simulink model "gm_parallel_min_cost_function_vopt_6phase"  (R2022a)
settings: Solver=FixedStepDiscrete  StartTime=0.0  StopTime=10.0  RelTol=1e-3
undefined symbols (not defined in the file or in its folder): f_c
libraries: hdlmdlgenlib x80
(part 2 of 3)

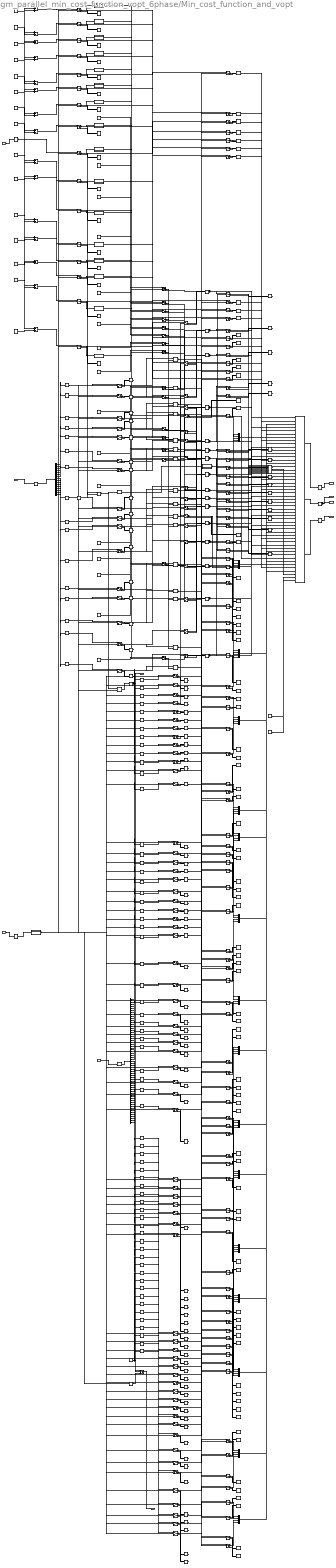
== system gm_parallel_min_cost_function_vopt_6phase/Min_cost_function_and_vopt ==
  Index_in : Inport  OutDataTypeStr=int32  PortDimensions=1  SampleTime=1e-08
  valid_in : Inport  Port=2  OutDataTypeStr=boolean  PortDimensions=1  SampleTime=1e-08
  J_in : Inport  Port=3  OutDataTypeStr=fixdt(1, 20, 11)  PortDimensions=[16]  SampleTime=1e-08
  phase_voltages_per_switching_state_in : Inport  Port=4  OutDataTypeStr=fixdt(1, 24, 11)  PortDimensions=[64]  SampleTime=1e-08
  Add{,1..14} (15 alike) : Sum  AccumDataTypeStr=fixdt(1, 33, 0)  OutDataTypeStr=fixdt(1, 33, 0)  SampleTime=1e-08
  Compare To Constant : Subsystem  mask(Compare To Constant){relop=<=, const=double(1), OutDataTypeStr=boolean, ZeroCross=on}
      mask prompts: relop "Simulink:masks:Operator_MP"; const "Simulink:masks:ConstantValue_MP"; OutDataTypeStr "Simulink:masks:OutputDataType_MP"; ZeroCross "Simulink:masks:EnableZerocrossingDetection_MP"
      mask help: Simulink:masks:CompareToConstant_MD
      mask init:
      | OutDataTypeStr = 'boolean';
      | ZeroCross = 'on';
      | blkName = 'parallel_min_cost_function_vopt_6phase/Min_cost_function_and_vopt/Compare\nTo Constant';
      | const = double(1);
      | const_str = '1';
      | const_val = double(1);
      | relop = '<=';
      | setValue = 'boolean';
      | str = '<= 1';
      mask TypeOptions relop: == | ~= | < | <= | >= | >
      mask TypeOptions OutDataTypeStr: Simulink:masks:uint8 | Simulink:masks:boolean
      mask Callback ZeroCross: sl('zeroCrossEnable', gcbh);
      mask Display: disp(str)
  Compare To Constant1 : Subsystem  mask(Compare To Constant){relop=<=, const=double(5), OutDataTypeStr=boolean, ZeroCross=on}
      mask prompts: relop "Simulink:masks:Operator_MP"; const "Simulink:masks:ConstantValue_MP"; OutDataTypeStr "Simulink:masks:OutputDataType_MP"; ZeroCross "Simulink:masks:EnableZerocrossingDetection_MP"
      mask help: Simulink:masks:CompareToConstant_MD
      mask init:
      | OutDataTypeStr = 'boolean';
      | ZeroCross = 'on';
      | blkName = 'parallel_min_cost_function_vopt_6phase/Min_cost_function_and_vopt/Compare\nTo Constant1';
      | const = double(5);
      | const_str = '5';
      | const_val = double(5);
      | relop = '<=';
      | setValue = 'boolean';
      | str = '<= 5';
      mask TypeOptions relop: == | ~= | < | <= | >= | >
      mask TypeOptions OutDataTypeStr: Simulink:masks:uint8 | Simulink:masks:boolean
      mask Callback ZeroCross: sl('zeroCrossEnable', gcbh);
      mask Display: disp(str)
  Compare To Constant10 : Subsystem  mask(Compare To Constant){relop=<=, const=double(41), OutDataTypeStr=boolean, ZeroCross=on}
      mask prompts: relop "Simulink:masks:Operator_MP"; const "Simulink:masks:ConstantValue_MP"; OutDataTypeStr "Simulink:masks:OutputDataType_MP"; ZeroCross "Simulink:masks:EnableZerocrossingDetection_MP"
      mask help: Simulink:masks:CompareToConstant_MD
      mask init:
      | OutDataTypeStr = 'boolean';
      | ZeroCross = 'on';
      | blkName = 'parallel_min_cost_function_vopt_6phase/Min_cost_function_and_vopt/Compare\nTo Constant10';
      | const = double(41);
      | const_str = '41';
      | const_val = double(41);
      | relop = '<=';
      | setValue = 'boolean';
      | str = '<= 41';
      mask TypeOptions relop: == | ~= | < | <= | >= | >
      mask TypeOptions OutDataTypeStr: Simulink:masks:uint8 | Simulink:masks:boolean
      mask Callback ZeroCross: sl('zeroCrossEnable', gcbh);
      mask Display: disp(str)
  Compare To Constant11 : Subsystem  mask(Compare To Constant){relop=<=, const=double(45), OutDataTypeStr=boolean, ZeroCross=on}
      mask prompts: relop "Simulink:masks:Operator_MP"; const "Simulink:masks:ConstantValue_MP"; OutDataTypeStr "Simulink:masks:OutputDataType_MP"; ZeroCross "Simulink:masks:EnableZerocrossingDetection_MP"
      mask help: Simulink:masks:CompareToConstant_MD
      mask init:
      | OutDataTypeStr = 'boolean';
      | ZeroCross = 'on';
      | blkName = 'parallel_min_cost_function_vopt_6phase/Min_cost_function_and_vopt/Compare\nTo Constant11';
      | const = double(45);
      | const_str = '45';
      | const_val = double(45);
      | relop = '<=';
      | setValue = 'boolean';
      | str = '<= 45';
      mask TypeOptions relop: == | ~= | < | <= | >= | >
      mask TypeOptions OutDataTypeStr: Simulink:masks:uint8 | Simulink:masks:boolean
      mask Callback ZeroCross: sl('zeroCrossEnable', gcbh);
      mask Display: disp(str)
  Compare To Constant12 : Subsystem  mask(Compare To Constant){relop=<=, const=double(49), OutDataTypeStr=boolean, ZeroCross=on}
      mask prompts: relop "Simulink:masks:Operator_MP"; const "Simulink:masks:ConstantValue_MP"; OutDataTypeStr "Simulink:masks:OutputDataType_MP"; ZeroCross "Simulink:masks:EnableZerocrossingDetection_MP"
      mask help: Simulink:masks:CompareToConstant_MD
      mask init:
      | OutDataTypeStr = 'boolean';
      | ZeroCross = 'on';
      | blkName = 'parallel_min_cost_function_vopt_6phase/Min_cost_function_and_vopt/Compare\nTo Constant12';
      | const = double(49);
      | const_str = '49';
      | const_val = double(49);
      | relop = '<=';
      | setValue = 'boolean';
      | str = '<= 49';
      mask TypeOptions relop: == | ~= | < | <= | >= | >
      mask TypeOptions OutDataTypeStr: Simulink:masks:uint8 | Simulink:masks:boolean
      mask Callback ZeroCross: sl('zeroCrossEnable', gcbh);
      mask Display: disp(str)
  Compare To Constant13 : Subsystem  mask(Compare To Constant){relop=<=, const=double(53), OutDataTypeStr=boolean, ZeroCross=on}
      mask prompts: relop "Simulink:masks:Operator_MP"; const "Simulink:masks:ConstantValue_MP"; OutDataTypeStr "Simulink:masks:OutputDataType_MP"; ZeroCross "Simulink:masks:EnableZerocrossingDetection_MP"
      mask help: Simulink:masks:CompareToConstant_MD
      mask init:
      | OutDataTypeStr = 'boolean';
      | ZeroCross = 'on';
      | blkName = 'parallel_min_cost_function_vopt_6phase/Min_cost_function_and_vopt/Compare\nTo Constant13';
      | const = double(53);
      | const_str = '53';
      | const_val = double(53);
      | relop = '<=';
      | setValue = 'boolean';
      | str = '<= 53';
      mask TypeOptions relop: == | ~= | < | <= | >= | >
      mask TypeOptions OutDataTypeStr: Simulink:masks:uint8 | Simulink:masks:boolean
      mask Callback ZeroCross: sl('zeroCrossEnable', gcbh);
      mask Display: disp(str)
  Compare To Constant14 : Subsystem  mask(Compare To Constant){relop=<=, const=double(57), OutDataTypeStr=boolean, ZeroCross=on}
      mask prompts: relop "Simulink:masks:Operator_MP"; const "Simulink:masks:ConstantValue_MP"; OutDataTypeStr "Simulink:masks:OutputDataType_MP"; ZeroCross "Simulink:masks:EnableZerocrossingDetection_MP"
      mask help: Simulink:masks:CompareToConstant_MD
      mask init:
      | OutDataTypeStr = 'boolean';
      | ZeroCross = 'on';
      | blkName = 'parallel_min_cost_function_vopt_6phase/Min_cost_function_and_vopt/Compare\nTo Constant14';
      | const = double(57);
      | const_str = '57';
      | const_val = double(57);
      | relop = '<=';
      | setValue = 'boolean';
      | str = '<= 57';
      mask TypeOptions relop: == | ~= | < | <= | >= | >
      mask TypeOptions OutDataTypeStr: Simulink:masks:uint8 | Simulink:masks:boolean
      mask Callback ZeroCross: sl('zeroCrossEnable', gcbh);
      mask Display: disp(str)
  Compare To Constant15 : Subsystem  mask(Compare To Constant){relop=<=, const=double(61), OutDataTypeStr=boolean, ZeroCross=on}
      mask prompts: relop "Simulink:masks:Operator_MP"; const "Simulink:masks:ConstantValue_MP"; OutDataTypeStr "Simulink:masks:OutputDataType_MP"; ZeroCross "Simulink:masks:EnableZerocrossingDetection_MP"
      mask help: Simulink:masks:CompareToConstant_MD
      mask init:
      | OutDataTypeStr = 'boolean';
      | ZeroCross = 'on';
      | blkName = 'parallel_min_cost_function_vopt_6phase/Min_cost_function_and_vopt/Compare\nTo Constant15';
      | const = double(61);
      | const_str = '61';
      | const_val = double(61);
      | relop = '<=';
      | setValue = 'boolean';
      | str = '<= 61';
      mask TypeOptions relop: == | ~= | < | <= | >= | >
      mask TypeOptions OutDataTypeStr: Simulink:masks:uint8 | Simulink:masks:boolean
      mask Callback ZeroCross: sl('zeroCrossEnable', gcbh);
      mask Display: disp(str)
  Compare To Constant2 : Subsystem  mask(Compare To Constant){relop=<=, const=double(9), OutDataTypeStr=boolean, ZeroCross=on}
      mask prompts: relop "Simulink:masks:Operator_MP"; const "Simulink:masks:ConstantValue_MP"; OutDataTypeStr "Simulink:masks:OutputDataType_MP"; ZeroCross "Simulink:masks:EnableZerocrossingDetection_MP"
      mask help: Simulink:masks:CompareToConstant_MD
      mask init:
      | OutDataTypeStr = 'boolean';
      | ZeroCross = 'on';
      | blkName = 'parallel_min_cost_function_vopt_6phase/Min_cost_function_and_vopt/Compare\nTo Constant2';
      | const = double(9);
      | const_str = '9';
      | const_val = double(9);
      | relop = '<=';
      | setValue = 'boolean';
      | str = '<= 9';
      mask TypeOptions relop: == | ~= | < | <= | >= | >
      mask TypeOptions OutDataTypeStr: Simulink:masks:uint8 | Simulink:masks:boolean
      mask Callback ZeroCross: sl('zeroCrossEnable', gcbh);
      mask Display: disp(str)
  Compare To Constant3 : Subsystem  mask(Compare To Constant){relop=<=, const=double(13), OutDataTypeStr=boolean, ZeroCross=on}
      mask prompts: relop "Simulink:masks:Operator_MP"; const "Simulink:masks:ConstantValue_MP"; OutDataTypeStr "Simulink:masks:OutputDataType_MP"; ZeroCross "Simulink:masks:EnableZerocrossingDetection_MP"
      mask help: Simulink:masks:CompareToConstant_MD
      mask init:
      | OutDataTypeStr = 'boolean';
      | ZeroCross = 'on';
      | blkName = 'parallel_min_cost_function_vopt_6phase/Min_cost_function_and_vopt/Compare\nTo Constant3';
      | const = double(13);
      | const_str = '13';
      | const_val = double(13);
      | relop = '<=';
      | setValue = 'boolean';
      | str = '<= 13';
      mask TypeOptions relop: == | ~= | < | <= | >= | >
      mask TypeOptions OutDataTypeStr: Simulink:masks:uint8 | Simulink:masks:boolean
      mask Callback ZeroCross: sl('zeroCrossEnable', gcbh);
      mask Display: disp(str)
  Compare To Constant4 : Subsystem  mask(Compare To Constant){relop=<=, const=double(17), OutDataTypeStr=boolean, ZeroCross=on}
      mask prompts: relop "Simulink:masks:Operator_MP"; const "Simulink:masks:ConstantValue_MP"; OutDataTypeStr "Simulink:masks:OutputDataType_MP"; ZeroCross "Simulink:masks:EnableZerocrossingDetection_MP"
      mask help: Simulink:masks:CompareToConstant_MD
      mask init:
      | OutDataTypeStr = 'boolean';
      | ZeroCross = 'on';
      | blkName = 'parallel_min_cost_function_vopt_6phase/Min_cost_function_and_vopt/Compare\nTo Constant4';
      | const = double(17);
      | const_str = '17';
      | const_val = double(17);
      | relop = '<=';
      | setValue = 'boolean';
      | str = '<= 17';
      mask TypeOptions relop: == | ~= | < | <= | >= | >
      mask TypeOptions OutDataTypeStr: Simulink:masks:uint8 | Simulink:masks:boolean
      mask Callback ZeroCross: sl('zeroCrossEnable', gcbh);
      mask Display: disp(str)
  Compare To Constant5 : Subsystem  mask(Compare To Constant){relop=<=, const=double(21), OutDataTypeStr=boolean, ZeroCross=on}
      mask prompts: relop "Simulink:masks:Operator_MP"; const "Simulink:masks:ConstantValue_MP"; OutDataTypeStr "Simulink:masks:OutputDataType_MP"; ZeroCross "Simulink:masks:EnableZerocrossingDetection_MP"
      mask help: Simulink:masks:CompareToConstant_MD
      mask init:
      | OutDataTypeStr = 'boolean';
      | ZeroCross = 'on';
      | blkName = 'parallel_min_cost_function_vopt_6phase/Min_cost_function_and_vopt/Compare\nTo Constant5';
      | const = double(21);
      | const_str = '21';
      | const_val = double(21);
      | relop = '<=';
      | setValue = 'boolean';
      | str = '<= 21';
      mask TypeOptions relop: == | ~= | < | <= | >= | >
      mask TypeOptions OutDataTypeStr: Simulink:masks:uint8 | Simulink:masks:boolean
      mask Callback ZeroCross: sl('zeroCrossEnable', gcbh);
      mask Display: disp(str)
  Compare To Constant6 : Subsystem  mask(Compare To Constant){relop=<=, const=double(25), OutDataTypeStr=boolean, ZeroCross=on}
      mask prompts: relop "Simulink:masks:Operator_MP"; const "Simulink:masks:ConstantValue_MP"; OutDataTypeStr "Simulink:masks:OutputDataType_MP"; ZeroCross "Simulink:masks:EnableZerocrossingDetection_MP"
      mask help: Simulink:masks:CompareToConstant_MD
      mask init:
      | OutDataTypeStr = 'boolean';
      | ZeroCross = 'on';
      | blkName = 'parallel_min_cost_function_vopt_6phase/Min_cost_function_and_vopt/Compare\nTo Constant6';
      | const = double(25);
      | const_str = '25';
      | const_val = double(25);
      | relop = '<=';
      | setValue = 'boolean';
      | str = '<= 25';
      mask TypeOptions relop: == | ~= | < | <= | >= | >
      mask TypeOptions OutDataTypeStr: Simulink:masks:uint8 | Simulink:masks:boolean
      mask Callback ZeroCross: sl('zeroCrossEnable', gcbh);
      mask Display: disp(str)
  Compare To Constant7 : Subsystem  mask(Compare To Constant){relop=<=, const=double(29), OutDataTypeStr=boolean, ZeroCross=on}
      mask prompts: relop "Simulink:masks:Operator_MP"; const "Simulink:masks:ConstantValue_MP"; OutDataTypeStr "Simulink:masks:OutputDataType_MP"; ZeroCross "Simulink:masks:EnableZerocrossingDetection_MP"
      mask help: Simulink:masks:CompareToConstant_MD
      mask init:
      | OutDataTypeStr = 'boolean';
      | ZeroCross = 'on';
      | blkName = 'parallel_min_cost_function_vopt_6phase/Min_cost_function_and_vopt/Compare\nTo Constant7';
      | const = double(29);
      | const_str = '29';
      | const_val = double(29);
      | relop = '<=';
      | setValue = 'boolean';
      | str = '<= 29';
      mask TypeOptions relop: == | ~= | < | <= | >= | >
      mask TypeOptions OutDataTypeStr: Simulink:masks:uint8 | Simulink:masks:boolean
      mask Callback ZeroCross: sl('zeroCrossEnable', gcbh);
      mask Display: disp(str)
  Compare To Constant8 : Subsystem  mask(Compare To Constant){relop=<=, const=double(33), OutDataTypeStr=boolean, ZeroCross=on}
      mask prompts: relop "Simulink:masks:Operator_MP"; const "Simulink:masks:ConstantValue_MP"; OutDataTypeStr "Simulink:masks:OutputDataType_MP"; ZeroCross "Simulink:masks:EnableZerocrossingDetection_MP"
      mask help: Simulink:masks:CompareToConstant_MD
      mask init:
      | OutDataTypeStr = 'boolean';
      | ZeroCross = 'on';
      | blkName = 'parallel_min_cost_function_vopt_6phase/Min_cost_function_and_vopt/Compare\nTo Constant8';
      | const = double(33);
      | const_str = '33';
      | const_val = double(33);
      | relop = '<=';
      | setValue = 'boolean';
      | str = '<= 33';
      mask TypeOptions relop: == | ~= | < | <= | >= | >
      mask TypeOptions OutDataTypeStr: Simulink:masks:uint8 | Simulink:masks:boolean
      mask Callback ZeroCross: sl('zeroCrossEnable', gcbh);
      mask Display: disp(str)
  Compare To Constant9 : Subsystem  mask(Compare To Constant){relop=<=, const=double(37), OutDataTypeStr=boolean, ZeroCross=on}
      mask prompts: relop "Simulink:masks:Operator_MP"; const "Simulink:masks:ConstantValue_MP"; OutDataTypeStr "Simulink:masks:OutputDataType_MP"; ZeroCross "Simulink:masks:EnableZerocrossingDetection_MP"
      mask help: Simulink:masks:CompareToConstant_MD
      mask init:
      | OutDataTypeStr = 'boolean';
      | ZeroCross = 'on';
      | blkName = 'parallel_min_cost_function_vopt_6phase/Min_cost_function_and_vopt/Compare\nTo Constant9';
      | const = double(37);
      | const_str = '37';
      | const_val = double(37);
      | relop = '<=';
      | setValue = 'boolean';
      | str = '<= 37';
      mask TypeOptions relop: == | ~= | < | <= | >= | >
      mask TypeOptions OutDataTypeStr: Simulink:masks:uint8 | Simulink:masks:boolean
      mask Callback ZeroCross: sl('zeroCrossEnable', gcbh);
      mask Display: disp(str)
  Constant{,3..17} (16 alike) : Constant  Value=250  OutDataTypeStr=fixdt(1, 20, 11)  SampleTime=1e-08
  Constant1 : Constant  Value=4  OutDataTypeStr=int32  SampleTime=1e-08
  Constant18 : Constant  Value=4  OutDataTypeStr=int32  SampleTime=1e-08
  Constant19 : Constant  Value=8  OutDataTypeStr=int32  SampleTime=1e-08
  Constant2 : Constant  Value=0  OutDataTypeStr=boolean  SampleTime=1e-08
  Constant20 : Constant  Value=12  OutDataTypeStr=int32  SampleTime=1e-08
  Constant21 : Constant  Value=16  OutDataTypeStr=int32  SampleTime=1e-08
  Constant22 : Constant  Value=20  OutDataTypeStr=int32  SampleTime=1e-08
  Constant23 : Constant  Value=24  OutDataTypeStr=int32  SampleTime=1e-08
  Constant24 : Constant  Value=28  OutDataTypeStr=int32  SampleTime=1e-08
  Constant25 : Constant  Value=32  OutDataTypeStr=int32  SampleTime=1e-08
  Constant26 : Constant  Value=36  OutDataTypeStr=int32  SampleTime=1e-08
  Constant27 : Constant  Value=40  OutDataTypeStr=int32  SampleTime=1e-08
  Constant28 : Constant  Value=44  OutDataTypeStr=int32  SampleTime=1e-08
  Constant29 : Constant  Value=48  OutDataTypeStr=int32  SampleTime=1e-08
  Constant30 : Constant  Value=52  OutDataTypeStr=int32  SampleTime=1e-08
  Constant31 : Constant  Value=56  OutDataTypeStr=int32  SampleTime=1e-08
  Constant32 : Constant  Value=60  OutDataTypeStr=int32  SampleTime=1e-08
  Constant33 : Constant  Value=0  OutDataTypeStr=fixdt(1, 20, 11)  SampleTime=1e-08
  Constant34 : Constant  Value="repmat(0,[4  1])"  OutDataTypeStr=fixdt(1, 24, 11)  SampleTime=1e-08
  Delay{,1..5,7..8,12..22,25..26,34..43,46,49..50,58..67,72..73,81..90,95..96,104..113,118..119,127..136,141..142,150..159,164..165,173..182,191..200,205..206,214..223,228..229,237..246,251..252,260..269,274..275,283..292,297..298,302..303,311..320,325..326,334..343,348..349,357..366,371..386} (216 alike) : Delay  DelayLength=double(1)  InitialCondition=0  SampleTime=1e-08
  Delay16_out1_0_wire : hdlmdlgenlib/Buffer
      settings: SourceProductBaseCode=SL
  Delay16_out1_10_wire : hdlmdlgenlib/Buffer
      settings: SourceProductBaseCode=SL
  Delay16_out1_11_wire : hdlmdlgenlib/Buffer
      settings: SourceProductBaseCode=SL
  Delay16_out1_12_wire : hdlmdlgenlib/Buffer
      settings: SourceProductBaseCode=SL
  Delay16_out1_13_wire : hdlmdlgenlib/Buffer
      settings: SourceProductBaseCode=SL
  Delay16_out1_14_wire : hdlmdlgenlib/Buffer
      settings: SourceProductBaseCode=SL
  Delay16_out1_15_wire : hdlmdlgenlib/Buffer
      settings: SourceProductBaseCode=SL
  Delay16_out1_16_wire : hdlmdlgenlib/Buffer
      settings: SourceProductBaseCode=SL
  Delay16_out1_17_wire : hdlmdlgenlib/Buffer
      settings: SourceProductBaseCode=SL
  Delay16_out1_18_wire : hdlmdlgenlib/Buffer
      settings: SourceProductBaseCode=SL
  Delay16_out1_19_wire : hdlmdlgenlib/Buffer
      settings: SourceProductBaseCode=SL
  Delay16_out1_1_wire : hdlmdlgenlib/Buffer
      settings: SourceProductBaseCode=SL
  Delay16_out1_20_wire : hdlmdlgenlib/Buffer
      settings: SourceProductBaseCode=SL
  Delay16_out1_21_wire : hdlmdlgenlib/Buffer
      settings: SourceProductBaseCode=SL
  Delay16_out1_22_wire : hdlmdlgenlib/Buffer
      settings: SourceProductBaseCode=SL
  Delay16_out1_23_wire : hdlmdlgenlib/Buffer
      settings: SourceProductBaseCode=SL
  Delay16_out1_24_wire : hdlmdlgenlib/Buffer
      settings: SourceProductBaseCode=SL
  Delay16_out1_25_wire : hdlmdlgenlib/Buffer
      settings: SourceProductBaseCode=SL
  Delay16_out1_26_wire : hdlmdlgenlib/Buffer
      settings: SourceProductBaseCode=SL
  Delay16_out1_27_wire : hdlmdlgenlib/Buffer
      settings: SourceProductBaseCode=SL
  Delay16_out1_28_wire : hdlmdlgenlib/Buffer
      settings: SourceProductBaseCode=SL
  Delay16_out1_29_wire : hdlmdlgenlib/Buffer
      settings: SourceProductBaseCode=SL
  Delay16_out1_2_wire : hdlmdlgenlib/Buffer
      settings: SourceProductBaseCode=SL
  Delay16_out1_30_wire : hdlmdlgenlib/Buffer
      settings: SourceProductBaseCode=SL
  Delay16_out1_31_wire : hdlmdlgenlib/Buffer
      settings: SourceProductBaseCode=SL
  Delay16_out1_32_wire : hdlmdlgenlib/Buffer
      settings: SourceProductBaseCode=SL
  Delay16_out1_33_wire : hdlmdlgenlib/Buffer
      settings: SourceProductBaseCode=SL
  Delay16_out1_34_wire : hdlmdlgenlib/Buffer
      settings: SourceProductBaseCode=SL
  Delay16_out1_35_wire : hdlmdlgenlib/Buffer
      settings: SourceProductBaseCode=SL
  Delay16_out1_36_wire : hdlmdlgenlib/Buffer
      settings: SourceProductBaseCode=SL
  Delay16_out1_37_wire : hdlmdlgenlib/Buffer
      settings: SourceProductBaseCode=SL
  Delay16_out1_38_wire : hdlmdlgenlib/Buffer
      settings: SourceProductBaseCode=SL
  Delay16_out1_39_wire : hdlmdlgenlib/Buffer
      settings: SourceProductBaseCode=SL
  Delay16_out1_3_wire : hdlmdlgenlib/Buffer
      settings: SourceProductBaseCode=SL
  Delay16_out1_40_wire : hdlmdlgenlib/Buffer
      settings: SourceProductBaseCode=SL
  Delay16_out1_41_wire : hdlmdlgenlib/Buffer
      settings: SourceProductBaseCode=SL
  Delay16_out1_42_wire : hdlmdlgenlib/Buffer
      settings: SourceProductBaseCode=SL
  Delay16_out1_43_wire : hdlmdlgenlib/Buffer
      settings: SourceProductBaseCode=SL
  Delay16_out1_44_wire : hdlmdlgenlib/Buffer
      settings: SourceProductBaseCode=SL
  Delay16_out1_45_wire : hdlmdlgenlib/Buffer
      settings: SourceProductBaseCode=SL
  Delay16_out1_46_wire : hdlmdlgenlib/Buffer
      settings: SourceProductBaseCode=SL
  Delay16_out1_47_wire : hdlmdlgenlib/Buffer
      settings: SourceProductBaseCode=SL
  Delay16_out1_48_wire : hdlmdlgenlib/Buffer
      settings: SourceProductBaseCode=SL
  Delay16_out1_49_wire : hdlmdlgenlib/Buffer
      settings: SourceProductBaseCode=SL
  Delay16_out1_4_wire : hdlmdlgenlib/Buffer
      settings: SourceProductBaseCode=SL
  Delay16_out1_50_wire : hdlmdlgenlib/Buffer
      settings: SourceProductBaseCode=SL
  Delay16_out1_51_wire : hdlmdlgenlib/Buffer
      settings: SourceProductBaseCode=SL
  Delay16_out1_52_wire : hdlmdlgenlib/Buffer
      settings: SourceProductBaseCode=SL
  Delay16_out1_53_wire : hdlmdlgenlib/Buffer
      settings: SourceProductBaseCode=SL
  Delay16_out1_54_wire : hdlmdlgenlib/Buffer
      settings: SourceProductBaseCode=SL
  Delay16_out1_55_wire : hdlmdlgenlib/Buffer
      settings: SourceProductBaseCode=SL
  Delay16_out1_56_wire : hdlmdlgenlib/Buffer
      settings: SourceProductBaseCode=SL
  Delay16_out1_57_wire : hdlmdlgenlib/Buffer
      settings: SourceProductBaseCode=SL
  Delay16_out1_58_wire : hdlmdlgenlib/Buffer
      settings: SourceProductBaseCode=SL
  Delay16_out1_59_wire : hdlmdlgenlib/Buffer
      settings: SourceProductBaseCode=SL
  Delay16_out1_5_wire : hdlmdlgenlib/Buffer
      settings: SourceProductBaseCode=SL
  Delay16_out1_60_wire : hdlmdlgenlib/Buffer
      settings: SourceProductBaseCode=SL
  Delay16_out1_61_wire : hdlmdlgenlib/Buffer
      settings: SourceProductBaseCode=SL
  Delay16_out1_62_wire : hdlmdlgenlib/Buffer
      settings: SourceProductBaseCode=SL
  Delay16_out1_63_wire : hdlmdlgenlib/Buffer
      settings: SourceProductBaseCode=SL
  Delay16_out1_6_wire : hdlmdlgenlib/Buffer
      settings: SourceProductBaseCode=SL
  Delay16_out1_7_wire : hdlmdlgenlib/Buffer
      settings: SourceProductBaseCode=SL
  Delay16_out1_8_wire : hdlmdlgenlib/Buffer
      settings: SourceProductBaseCode=SL
  Delay16_out1_9_wire : hdlmdlgenlib/Buffer
      settings: SourceProductBaseCode=SL
  Delay23 : Delay  DelayLength=double(3)  InitialCondition=0  SampleTime=1e-08
  Delay24 : Delay  DelayLength=double(3)  InitialCondition=0  SampleTime=1e-08
  Delay7_out1_0_wire : hdlmdlgenlib/Buffer
      settings: SourceProductBaseCode=SL
  Delay7_out1_10_wire : hdlmdlgenlib/Buffer
      settings: SourceProductBaseCode=SL
  Delay7_out1_11_wire : hdlmdlgenlib/Buffer
      settings: SourceProductBaseCode=SL
  Delay7_out1_12_wire : hdlmdlgenlib/Buffer
      settings: SourceProductBaseCode=SL
  Delay7_out1_13_wire : hdlmdlgenlib/Buffer
      settings: SourceProductBaseCode=SL
  Delay7_out1_14_wire : hdlmdlgenlib/Buffer
      settings: SourceProductBaseCode=SL
  Delay7_out1_15_wire : hdlmdlgenlib/Buffer
      settings: SourceProductBaseCode=SL
  Delay7_out1_1_wire : hdlmdlgenlib/Buffer
      settings: SourceProductBaseCode=SL
  Delay7_out1_2_wire : hdlmdlgenlib/Buffer
      settings: SourceProductBaseCode=SL
  Delay7_out1_3_wire : hdlmdlgenlib/Buffer
      settings: SourceProductBaseCode=SL
  Delay7_out1_4_wire : hdlmdlgenlib/Buffer
      settings: SourceProductBaseCode=SL
  Delay7_out1_5_wire : hdlmdlgenlib/Buffer
      settings: SourceProductBaseCode=SL
  Delay7_out1_6_wire : hdlmdlgenlib/Buffer
      settings: SourceProductBaseCode=SL
  Delay7_out1_7_wire : hdlmdlgenlib/Buffer
      settings: SourceProductBaseCode=SL
  Delay7_out1_8_wire : hdlmdlgenlib/Buffer
      settings: SourceProductBaseCode=SL
  Delay7_out1_9_wire : hdlmdlgenlib/Buffer
      settings: SourceProductBaseCode=SL
  Detect Rise Positive : Subsystem  mask(Detect Rise Positive){vinit=double(0), InputProcessing=Elements as channels (sample based), OutDataTypeStr=boolean}
      mask prompts: vinit "Simulink:masks:InitialCondition_MP"; InputProcessing "Simulink:masks:InputProcessing_MP"; OutDataTypeStr "Simulink:masks:OutputDataType_MP"
      mask help: Simulink:masks:DetectRisePositive_MD
      mask init:
      | InputProcessing = 'Elements as channels (sample based)';
      | OutDataTypeStr = 'boolean';
      | vinit = double(0);
      mask TypeOptions InputProcessing: Simulink:masks:ColumnsAsChannelsFrameBased | Simulink:masks:ElementsAsChannelsSampleBased
      mask TypeOptions OutDataTypeStr: Simulink:masks:uint8 | Simulink:masks:boolean
      mask Display: fprintf('U > 0\n&  NOT\nU/z > 0')
  Detect Rise Positive1 : Subsystem  mask(Detect Rise Positive){vinit=double(0), InputProcessing=Elements as channels (sample based), OutDataTypeStr=boolean}
      mask prompts: vinit "Simulink:masks:InitialCondition_MP"; InputProcessing "Simulink:masks:InputProcessing_MP"; OutDataTypeStr "Simulink:masks:OutputDataType_MP"
      mask help: Simulink:masks:DetectRisePositive_MD
      mask init:
      | InputProcessing = 'Elements as channels (sample based)';
      | OutDataTypeStr = 'boolean';
      | vinit = double(0);
      mask TypeOptions InputProcessing: Simulink:masks:ColumnsAsChannelsFrameBased | Simulink:masks:ElementsAsChannelsSampleBased
      mask TypeOptions OutDataTypeStr: Simulink:masks:uint8 | Simulink:masks:boolean
      mask Display: fprintf('U > 0\n&  NOT\nU/z > 0')
  Logical Operator : Logic  AllPortsSameDT=off  OutDataTypeStr=boolean  SampleTime=1e-08
  MATLAB Function : Subsystem
  MinMax : MinMax  Inputs=16
  Relational Operator{,2..16} (16 alike) : RelationalOperator  Operator=<=  OutDataTypeStr=boolean  SampleTime=1e-08  InputSameDT=off
  Relational Operator1 : RelationalOperator  Operator===  OutDataTypeStr=boolean  SampleTime=1e-08  InputSameDT=off
  Switch{,1,8..9,20..21,27..28,34..35,41..42,48..49,55..56,62..63,69..70,76..77,83..84,90..91,97..98,104..105,111..112} (32 alike) : Switch  Criteria=u2 > Threshold  Threshold=double(0)  OutDataTypeStr=fixdt(1, 20, 11)  SampleTime=1e-08  SaturateOnIntegerOverflow=off  InputSameDT=off
  Switch{2,10,15,22,29,36,43,50,57,64,71,78,85,92,99,106} (16 alike) : Switch  Criteria=u2 > Threshold  Threshold=double(0)  OutDataTypeStr=int32  SampleTime=1e-08  SaturateOnIntegerOverflow=off  InputSameDT=off
  Switch{3..6,11..14,16..19,23..26,30..33,37..40,44..47,51..54,58..61,65..68,72..75,79..82,86..89,93..96,100..103,107..110} (64 alike) : Switch  Criteria=u2 > Threshold  Threshold=double(0)  OutDataTypeStr=fixdt(1, 24, 11)  SampleTime=1e-08  SaturateOnIntegerOverflow=off  InputSameDT=off
  Switch7 : Switch  Criteria=u2 > Threshold  Threshold=double(0)  OutDataTypeStr=boolean  SampleTime=1e-08  SaturateOnIntegerOverflow=off  InputSameDT=off
  Switch_on1 : Switch  Threshold=double(1)  OutDataTypeStr=int32  RndMeth=Simplest  SampleTime=1e-08  SaturateOnIntegerOverflow=off  InputSameDT=off
  Switch_on{4,10,14,20,26,32,38,44,50,56,62,68,74,80,86,92,98..113} (32 alike) : Switch  Threshold=double(1)  OutDataTypeStr=fixdt(1, 20, 11)  RndMeth=Simplest  SampleTime=1e-08  SaturateOnIntegerOverflow=off  InputSameDT=off
  Switch_on{2..3,5..6,8..9,11..12,15..16,18..19,21..22,24..25,27..28,30..31,33..34,36..37,39..40,42..43,45..46,48..49,51..52,54..55,57..58,60..61,63..64,66..67,69..70,72..73,75..76,78..79,81..82,84..85,87..88,90..91,93..94,96..97} (64 alike) : Switch  Threshold=double(1)  OutDataTypeStr=fixdt(1, 24, 11)  RndMeth=Simplest  SampleTime=1e-08  SaturateOnIntegerOverflow=off  InputSameDT=off
  Switch_on{7,17,23,29,35,41,47,53,59,65,71,77,83,89,95} (15 alike) : Switch  Threshold=double(1)  OutDataTypeStr=fixdt(1, 33, 0)  RndMeth=Simplest  SampleTime=1e-08  SaturateOnIntegerOverflow=off  InputSameDT=off
  mux{,1..15} (16 alike) : Mux
  t : Demux  Outputs=16
  t1 : Demux  Outputs=64
  done : Outport  SampleTime=1e-08
  done_complete : Outport  Port=2  SampleTime=1e-08
  J_AXI : Outport  Port=3  SampleTime=1e-08
  Index : Outport  Port=4  SampleTime=1e-08
  voltages : Outport  Port=5  SampleTime=1e-08
  Index_AXI : Outport  Port=6  SampleTime=1e-08
  wires:
  Index_in/1 -> Delay8/1
  valid_in/1 -> Delay46/1
  J_in/1 -> Delay7/1
  phase_voltages_per_switching_state_in/1 -> Delay16/1
  Add/1 -> Switch_on7/1
  Add1/1 -> Switch_on17/1
  Add10/1 -> Switch_on71/1
  Add11/1 -> Switch_on77/1
  Add12/1 -> Switch_on83/1
  Add13/1 -> Switch_on89/1
  Add14/1 -> Switch_on95/1
  Add2/1 -> Switch_on23/1
  Add3/1 -> Switch_on29/1
  Add4/1 -> Switch_on35/1
  Add5/1 -> Switch_on41/1
  Add6/1 -> Switch_on47/1
  Add7/1 -> Switch_on53/1
  Add8/1 -> Switch_on59/1
  Add9/1 -> Switch_on65/1
  Compare To Constant/1(y) -> Switch/2
  Compare To Constant1/1(y) -> Switch8/2
  Compare To Constant10/1(y) -> Switch76/2
  Compare To Constant11/1(y) -> Switch83/2
  Compare To Constant12/1(y) -> Switch90/2
  Compare To Constant13/1(y) -> Switch97/2
  Compare To Constant14/1(y) -> Switch104/2
  Compare To Constant15/1(y) -> Switch111/2
  Compare To Constant2/1(y) -> Switch20/2
  Compare To Constant3/1(y) -> Switch27/2
  Compare To Constant4/1(y) -> Switch34/2
  Compare To Constant5/1(y) -> Switch41/2
  Compare To Constant6/1(y) -> Switch48/2
  Compare To Constant7/1(y) -> Switch55/2
  Compare To Constant8/1(y) -> Switch62/2
  Compare To Constant9/1(y) -> Switch69/2
  Constant/1 -> Switch/1
  Constant1/1 -> Relational Operator1/1
  Constant10/1 -> Switch62/1
  Constant11/1 -> Switch69/1
  Constant12/1 -> Switch76/1
  Constant13/1 -> Switch83/1
  Constant14/1 -> Switch90/1
  Constant15/1 -> Switch97/1
  Constant16/1 -> Switch104/1
  Constant17/1 -> Switch111/1
  Constant18/1 -> Add/2
  Constant19/1 -> Add1/2
  Constant2/1 -> Switch7/1
  Constant20/1 -> Add2/2
  Constant21/1 -> Add3/2
  Constant22/1 -> Add4/2
  Constant23/1 -> Add5/2
  Constant24/1 -> Add6/2
  Constant25/1 -> Add7/2
  Constant26/1 -> Add8/2
  Constant27/1 -> Add9/2
  Constant28/1 -> Add10/2
  Constant29/1 -> Add11/2
  Constant3/1 -> Switch8/1
  Constant30/1 -> Add12/2
  Constant31/1 -> Add13/2
  Constant32/1 -> Add14/2
  Constant33/1 -> MATLAB Function/50(J_default)
  Constant34/1 -> MATLAB Function/51(voltages_default)
  Constant4/1 -> Switch20/1
  Constant5/1 -> Switch27/1
  Constant6/1 -> Switch34/1
  Constant7/1 -> Switch41/1
  Constant8/1 -> Switch48/1
  Constant9/1 -> Switch55/1
  Delay/1 -> Switch_on98/1, Switch1/3, Switch/3, MATLAB Function/1(J_1)
  Delay1/1 -> Switch2/3
  Delay104/1 -> Switch_on26/3
  Delay105/1 -> Switch_on29/3
  Delay106/1 -> Switch_on30/3
  Delay107/1 -> Switch30/3
  Delay108/1 -> Switch_on31/3
  Delay109/1 -> Switch_on27/3
  Delay110/1 -> Switch_on28/3
  Delay111/1 -> Switch31/3
  Delay112/1 -> Switch32/3
  Delay113/1 -> Switch33/3
  Delay118/1 -> Switch_on105/1, Switch42/3, Switch41/3, MATLAB Function/16(J_6)
  Delay119/1 -> Switch36/3
  Delay12/1 -> J_AXI/1
  Delay127/1 -> Switch_on32/3
  Delay128/1 -> Switch_on35/3
  Delay129/1 -> Switch_on36/3
  Delay13/1 -> Index_AXI/1, Index/1
  Delay130/1 -> Switch37/3
  Delay131/1 -> Switch_on37/3
  Delay132/1 -> Switch_on33/3
  Delay133/1 -> Switch_on34/3
  Delay134/1 -> Switch38/3
  Delay135/1 -> Switch39/3
  Delay136/1 -> Switch40/3
  Delay14/1 -> voltages/1
  Delay141/1 -> Switch_on102/1, Switch49/3, Switch48/3, MATLAB Function/19(J_7)
  Delay142/1 -> Switch43/3
  Delay15/1 -> Detect Rise Positive1/1(U)
  Delay150/1 -> Switch_on38/3
  Delay151/1 -> Switch_on41/3
  Delay152/1 -> Switch_on42/3
  Delay153/1 -> Switch44/3
  Delay154/1 -> Switch_on43/3
  Delay155/1 -> Switch_on39/3
  Delay156/1 -> Switch_on40/3
  Delay157/1 -> Switch45/3
  Delay158/1 -> Switch46/3
  Delay159/1 -> Switch47/3
  Delay16/1 -> t1/1
  Delay164/1 -> Switch_on103/1, Switch56/3, Switch55/3, MATLAB Function/22(J_8)
  Delay165/1 -> Switch50/3
  Delay17/1 -> Switch_on4/3
  Delay173/1 -> Switch_on44/3
  Delay174/1 -> Switch_on47/3
  Delay175/1 -> Switch_on48/3
  Delay176/1 -> Switch51/3
  Delay177/1 -> Switch_on49/3
  Delay178/1 -> Switch_on45/3
  Delay179/1 -> Switch_on46/3
  Delay18/1 -> Switch_on1/3
  Delay180/1 -> Switch52/3
  Delay181/1 -> Switch53/3
  Delay182/1 -> Switch54/3
  Delay19/1 -> Switch_on2/3
  Delay191/1 -> Switch_on56/3
  Delay192/1 -> Switch_on59/3
  Delay193/1 -> Switch_on60/3
  Delay194/1 -> Switch65/3
  Delay195/1 -> Switch_on61/3
  Delay196/1 -> Switch_on57/3
  Delay197/1 -> Switch_on58/3
  Delay198/1 -> Switch66/3
  Delay199/1 -> Switch67/3
  Delay2/1 -> Switch3/3
  Delay20/1 -> Switch_on3/3
  Delay200/1 -> Switch68/3
  Delay205/1 -> Switch_on106/1, Switch77/3, Switch76/3, MATLAB Function/31(J_11)
  Delay206/1 -> Switch71/3
  Delay21/1 -> Switch_on5/3
  Delay214/1 -> Switch_on62/3
  Delay215/1 -> Switch_on65/3
  Delay216/1 -> Switch_on66/3
  Delay217/1 -> Switch72/3
  Delay218/1 -> Switch_on67/3
  Delay219/1 -> Switch_on63/3
  Delay22/1 -> Switch_on6/3
  Delay220/1 -> Switch_on64/3
  Delay221/1 -> Switch73/3
  Delay222/1 -> Switch74/3
  Delay223/1 -> Switch75/3
  Delay228/1 -> Switch_on107/1, Switch84/3, Switch83/3, MATLAB Function/34(J_12)
  Delay229/1 -> Switch78/3
  Delay23/1 -> Switch7/2, done_complete/1
  Delay237/1 -> Switch_on68/3
  Delay238/1 -> Switch_on71/3
  Delay239/1 -> Switch_on72/3
  Delay24/1 -> Switch7/3
  Delay240/1 -> Switch79/3
  Delay241/1 -> Switch_on73/3
  Delay242/1 -> Switch_on69/3
  Delay243/1 -> Switch_on70/3
  Delay244/1 -> Switch80/3
  Delay245/1 -> Switch81/3
  Delay246/1 -> Switch82/3
  Delay25/1 -> Switch_on99/1, Switch9/3, Switch8/3, MATLAB Function/4(J_2)
  Delay251/1 -> Switch_on112/1, Switch91/3, Switch90/3, MATLAB Function/37(J_13)
  Delay252/1 -> Switch85/3
  Delay26/1 -> Switch10/3
  Delay260/1 -> Switch_on74/3
  Delay261/1 -> Switch_on77/3
  Delay262/1 -> Switch_on78/3
  Delay263/1 -> Switch86/3
  Delay264/1 -> Switch_on79/3
  Delay265/1 -> Switch_on75/3
  Delay266/1 -> Switch_on76/3
  Delay267/1 -> Switch87/3
  Delay268/1 -> Switch88/3
  Delay269/1 -> Switch89/3
  Delay274/1 -> Switch_on108/1, Switch63/3, Switch62/3, MATLAB Function/25(J_9)
  Delay275/1 -> Switch57/3
  Delay283/1 -> Switch_on50/3
  Delay284/1 -> Switch_on53/3
  Delay285/1 -> Switch_on54/3
  Delay286/1 -> Switch58/3
  Delay287/1 -> Switch_on55/3
  Delay288/1 -> Switch_on51/3
  Delay289/1 -> Switch_on52/3
  Delay290/1 -> Switch59/3
  Delay291/1 -> Switch60/3
  Delay292/1 -> Switch61/3
  Delay297/1 -> Switch_on109/1, Switch70/3, Switch69/3, MATLAB Function/28(J_10)
  Delay298/1 -> Switch64/3
  Delay3/1 -> Switch4/3
  Delay302/1 -> Switch_on113/1, Switch98/3, Switch97/3, MATLAB Function/40(J_14)
  Delay303/1 -> Switch92/3
  Delay311/1 -> Switch_on80/3
  Delay312/1 -> Switch_on83/3
  Delay313/1 -> Switch_on84/3
  Delay314/1 -> Switch93/3
  Delay315/1 -> Switch_on85/3
  Delay316/1 -> Switch_on81/3
  Delay317/1 -> Switch_on82/3
  Delay318/1 -> Switch94/3
  Delay319/1 -> Switch95/3
  Delay320/1 -> Switch96/3
  Delay325/1 -> Switch_on110/1, Switch105/3, Switch104/3, MATLAB Function/43(J_15)
  Delay326/1 -> Switch99/3
  Delay334/1 -> Switch_on86/3
  Delay335/1 -> Switch_on89/3
  Delay336/1 -> Switch_on90/3
  Delay337/1 -> Switch100/3
  Delay338/1 -> Switch_on91/3
  Delay339/1 -> Switch_on87/3
  Delay34/1 -> Switch_on10/3
  Delay340/1 -> Switch_on88/3
  Delay341/1 -> Switch101/3
  Delay342/1 -> Switch102/3
  Delay343/1 -> Switch103/3
  Delay348/1 -> Switch_on111/1, Switch112/3, Switch111/3, MATLAB Function/46(J_16)
  Delay349/1 -> Switch106/3
  Delay35/1 -> Switch_on7/3
  Delay357/1 -> Switch_on92/3
  Delay358/1 -> Switch_on95/3
  Delay359/1 -> Switch_on96/3
  Delay36/1 -> Switch_on8/3
  Delay360/1 -> Switch107/3
  Delay361/1 -> Switch_on97/3
  Delay362/1 -> Switch_on93/3
  Delay363/1 -> Switch_on94/3
  Delay364/1 -> Switch108/3
  Delay365/1 -> Switch109/3
  Delay366/1 -> Switch110/3
  Delay37/1 -> Switch11/3
  Delay371/1 -> Switch_on98/3
  Delay372/1 -> Switch_on99/3
  Delay373/1 -> Switch_on100/3
  Delay374/1 -> Switch_on101/3
  Delay375/1 -> Switch_on104/3
  Delay376/1 -> Switch_on105/3
  Delay377/1 -> Switch_on102/3
  Delay378/1 -> Switch_on103/3
  Delay379/1 -> Switch_on108/3
  Delay38/1 -> Switch_on9/3
  Delay380/1 -> Switch_on109/3
  Delay381/1 -> Switch_on106/3
  Delay382/1 -> Switch_on107/3
  Delay383/1 -> Switch_on112/3
  Delay384/1 -> Switch_on113/3
  Delay385/1 -> Switch_on110/3
  Delay386/1 -> Switch_on111/3
  Delay39/1 -> Switch_on11/3
  Delay4/1 -> Switch5/3
  Delay40/1 -> Switch_on12/3
  Delay41/1 -> Switch12/3
  Delay42/1 -> Switch13/3
  Delay43/1 -> Switch14/3
  Delay46/1 -> Detect Rise Positive/1(U)
  Delay49/1 -> Switch_on100/1, Switch21/3, Switch20/3, MATLAB Function/7(J_3)
  Delay5/1 -> Switch6/3
  Delay50/1 -> Switch15/3
  Delay58/1 -> Switch_on14/3
  Delay59/1 -> Switch_on17/3
  Delay60/1 -> Switch_on18/3
  Delay61/1 -> Switch16/3
  Delay62/1 -> Switch_on19/3
  Delay63/1 -> Switch_on15/3
  Delay64/1 -> Switch_on16/3
  Delay65/1 -> Switch17/3
  Delay66/1 -> Switch18/3
  Delay67/1 -> Switch19/3
  Delay7/1 -> t/1
  Delay72/1 -> Switch_on101/1, Switch28/3, Switch27/3, MATLAB Function/10(J_4)
  Delay73/1 -> Switch22/3
  Delay8/1 -> Switch_on1/1, Add9/1, Add8/1, Add7/1, Add6/1, Add5/1, Add4/1, Add3/1, Add2/1, Add14/1, Add13/1, Add12/1, Add11/1, Add10/1, Add1/1, Add/1
  Delay81/1 -> Switch_on20/3
  Delay82/1 -> Switch_on23/3
  Delay83/1 -> Switch_on24/3
  Delay84/1 -> Switch23/3
  Delay85/1 -> Switch_on25/3
  Delay86/1 -> Switch_on21/3
  Delay87/1 -> Switch_on22/3
  Delay88/1 -> Switch24/3
  Delay89/1 -> Switch25/3
  Delay90/1 -> Switch26/3
  Delay95/1 -> Switch_on104/1, Switch35/3, Switch34/3, MATLAB Function/13(J_5)
  Delay96/1 -> Switch29/3
  Delay7_out1_0_wire/1 -> Switch_on4/1
  Delay7_out1_1_wire/1 -> Switch_on10/1
  Delay7_out1_2_wire/1 -> Switch_on14/1
  Delay7_out1_3_wire/1 -> Switch_on20/1
  Delay7_out1_4_wire/1 -> Switch_on26/1
  Delay7_out1_5_wire/1 -> Switch_on32/1
  Delay7_out1_6_wire/1 -> Switch_on38/1
  Delay7_out1_7_wire/1 -> Switch_on44/1
  Delay7_out1_8_wire/1 -> Switch_on50/1
  Delay7_out1_9_wire/1 -> Switch_on56/1
  Delay7_out1_10_wire/1 -> Switch_on62/1
  Delay7_out1_11_wire/1 -> Switch_on68/1
  Delay7_out1_12_wire/1 -> Switch_on74/1
  Delay7_out1_13_wire/1 -> Switch_on80/1
  Delay7_out1_14_wire/1 -> Switch_on86/1
  Delay7_out1_15_wire/1 -> Switch_on92/1
  Delay16_out1_0_wire/1 -> Switch_on2/1
  Delay16_out1_1_wire/1 -> Switch_on3/1
  Delay16_out1_2_wire/1 -> Switch_on5/1
  Delay16_out1_3_wire/1 -> Switch_on6/1
  Delay16_out1_4_wire/1 -> Switch_on8/1
  Delay16_out1_5_wire/1 -> Switch_on9/1
  Delay16_out1_6_wire/1 -> Switch_on11/1
  Delay16_out1_7_wire/1 -> Switch_on12/1
  Delay16_out1_8_wire/1 -> Switch_on18/1
  Delay16_out1_9_wire/1 -> Switch_on19/1
  Delay16_out1_10_wire/1 -> Switch_on15/1
  Delay16_out1_11_wire/1 -> Switch_on16/1
  Delay16_out1_12_wire/1 -> Switch_on24/1
  Delay16_out1_13_wire/1 -> Switch_on25/1
  Delay16_out1_14_wire/1 -> Switch_on21/1
  Delay16_out1_15_wire/1 -> Switch_on22/1
  Delay16_out1_16_wire/1 -> Switch_on30/1
  Delay16_out1_17_wire/1 -> Switch_on31/1
  Delay16_out1_18_wire/1 -> Switch_on27/1
  Delay16_out1_19_wire/1 -> Switch_on28/1
  Delay16_out1_20_wire/1 -> Switch_on36/1
  Delay16_out1_21_wire/1 -> Switch_on37/1
  Delay16_out1_22_wire/1 -> Switch_on33/1
  Delay16_out1_23_wire/1 -> Switch_on34/1
  Delay16_out1_24_wire/1 -> Switch_on42/1
  Delay16_out1_25_wire/1 -> Switch_on43/1
  Delay16_out1_26_wire/1 -> Switch_on39/1
  Delay16_out1_27_wire/1 -> Switch_on40/1
  Delay16_out1_28_wire/1 -> Switch_on48/1
  Delay16_out1_29_wire/1 -> Switch_on49/1
  Delay16_out1_30_wire/1 -> Switch_on45/1
  Delay16_out1_31_wire/1 -> Switch_on46/1
  Delay16_out1_32_wire/1 -> Switch_on54/1
  Delay16_out1_33_wire/1 -> Switch_on55/1
  Delay16_out1_34_wire/1 -> Switch_on51/1
  Delay16_out1_35_wire/1 -> Switch_on52/1
  Delay16_out1_36_wire/1 -> Switch_on60/1
  Delay16_out1_37_wire/1 -> Switch_on61/1
  Delay16_out1_38_wire/1 -> Switch_on57/1
  Delay16_out1_39_wire/1 -> Switch_on58/1
  Delay16_out1_40_wire/1 -> Switch_on66/1
  Delay16_out1_41_wire/1 -> Switch_on67/1
  Delay16_out1_42_wire/1 -> Switch_on63/1
  Delay16_out1_43_wire/1 -> Switch_on64/1
  Delay16_out1_44_wire/1 -> Switch_on72/1
  Delay16_out1_45_wire/1 -> Switch_on73/1
  Delay16_out1_46_wire/1 -> Switch_on69/1
  Delay16_out1_47_wire/1 -> Switch_on70/1
  Delay16_out1_48_wire/1 -> Switch_on78/1
  Delay16_out1_49_wire/1 -> Switch_on79/1
  Delay16_out1_50_wire/1 -> Switch_on75/1
  Delay16_out1_51_wire/1 -> Switch_on76/1
  Delay16_out1_52_wire/1 -> Switch_on84/1
  Delay16_out1_53_wire/1 -> Switch_on85/1
  Delay16_out1_54_wire/1 -> Switch_on81/1
  Delay16_out1_55_wire/1 -> Switch_on82/1
  Delay16_out1_56_wire/1 -> Switch_on90/1
  Delay16_out1_57_wire/1 -> Switch_on91/1
  Delay16_out1_58_wire/1 -> Switch_on87/1
  Delay16_out1_59_wire/1 -> Switch_on88/1
  Delay16_out1_60_wire/1 -> Switch_on96/1
  Delay16_out1_61_wire/1 -> Switch_on97/1
  Delay16_out1_62_wire/1 -> Switch_on93/1
  Delay16_out1_63_wire/1 -> Switch_on94/1
  Detect Rise Positive/1(Y) -> Switch_on97/2, Switch_on96/2, Switch_on95/2, Switch_on94/2, Switch_on93/2, Switch_on92/2, Switch_on91/2, Switch_on90/2, Switch_on9/2, Switch_on89/2, Switch_on88/2, Switch_on87/2, Switch_on86/2, Switch_on85/2, Switch_on84/2, Switch_on83/2, Switch_on82/2, Switch_on81/2, Switch_on80/2, Switch_on8/2, Switch_on79/2, Switch_on78/2, Switch_on77/2, Switch_on76/2, Switch_on75/2, Switch_on74/2, Switch_on73/2, Switch_on72/2, Switch_on71/2, Switch_on70/2, Switch_on7/2, Switch_on69/2, Switch_on68/2, Switch_on67/2, Switch_on66/2, Switch_on65/2, Switch_on64/2, Switch_on63/2, Switch_on62/2, Switch_on61/2, Switch_on60/2, Switch_on6/2, Switch_on59/2, Switch_on58/2, Switch_on57/2, Switch_on56/2, Switch_on55/2, Switch_on54/2, Switch_on53/2, Switch_on52/2, Switch_on51/2, Switch_on50/2, Switch_on5/2, Switch_on49/2, Switch_on48/2, Switch_on47/2, Switch_on46/2, Switch_on45/2, Switch_on44/2, Switch_on43/2, Switch_on42/2, Switch_on41/2, Switch_on40/2, Switch_on4/2, Switch_on39/2, Switch_on38/2, Switch_on37/2, Switch_on36/2, Switch_on35/2, Switch_on34/2, Switch_on33/2, Switch_on32/2, Switch_on31/2, Switch_on30/2, Switch_on3/2, Switch_on29/2, Switch_on28/2, Switch_on27/2, Switch_on26/2, Switch_on25/2, Switch_on24/2, Switch_on23/2, Switch_on22/2, Switch_on21/2, Switch_on20/2, Switch_on2/2, Switch_on19/2, Switch_on18/2, Switch_on17/2, Switch_on16/2, Switch_on15/2, Switch_on14/2, Switch_on12/2, Switch_on11/2, Switch_on10/2, Switch_on1/2, Logical Operator/2, Delay24/1
  Detect Rise Positive1/1(Y) -> Switch_on99/2, Switch_on98/2, Switch_on113/2, Switch_on112/2, Switch_on111/2, Switch_on110/2, Switch_on109/2, Switch_on108/2, Switch_on107/2, Switch_on106/2, Switch_on105/2, Switch_on104/2, Switch_on103/2, Switch_on102/2, Switch_on101/2, Switch_on100/2
  Logical Operator/1 -> Delay23/1
  MATLAB Function/1(J) -> Delay12/1
  MATLAB Function/2(Index) -> Delay13/1
  MATLAB Function/3(voltages) -> Delay14/1
  MinMax/1 -> MATLAB Function/49(min)
  mux/1 -> MATLAB Function/3(voltages_1)
  mux1/1 -> MATLAB Function/6(voltages_2)
  mux2/1 -> MATLAB Function/33(voltages_11)
  mux3/1 -> MATLAB Function/36(voltages_12)
  mux4/1 -> MATLAB Function/39(voltages_13)
  mux5/1 -> MATLAB Function/42(voltages_14)
  mux6/1 -> MATLAB Function/45(voltages_15)
  mux7/1 -> MATLAB Function/48(voltages_16)
  mux8/1 -> MATLAB Function/9(voltages_3)
  mux9/1 -> MATLAB Function/12(voltages_4)
  mux10/1 -> MATLAB Function/15(voltages_5)
  mux11/1 -> MATLAB Function/18(voltages_6)
  mux12/1 -> MATLAB Function/21(voltages_7)
  mux13/1 -> MATLAB Function/24(voltages_8)
  mux14/1 -> MATLAB Function/27(voltages_9)
  mux15/1 -> MATLAB Function/30(voltages_10)
  Relational Operator/1 -> Switch6/2, Switch5/2, Switch4/2, Switch3/2, Switch2/2, Switch1/2
  Relational Operator1/1 -> Logical Operator/1, Delay15/1
  Relational Operator10/1 -> Switch70/2, Switch68/2, Switch67/2, Switch66/2, Switch65/2, Switch64/2
  Relational Operator11/1 -> Switch77/2, Switch75/2, Switch74/2, Switch73/2, Switch72/2, Switch71/2
  Relational Operator12/1 -> Switch84/2, Switch82/2, Switch81/2, Switch80/2, Switch79/2, Switch78/2
  Relational Operator13/1 -> Switch91/2, Switch89/2, Switch88/2, Switch87/2, Switch86/2, Switch85/2
  Relational Operator14/1 -> Switch98/2, Switch96/2, Switch95/2, Switch94/2, Switch93/2, Switch92/2
  Relational Operator15/1 -> Switch99/2, Switch105/2, Switch103/2, Switch102/2, Switch101/2, Switch100/2
  Relational Operator16/1 -> Switch112/2, Switch110/2, Switch109/2, Switch108/2, Switch107/2, Switch106/2
  Relational Operator2/1 -> Switch9/2, Switch14/2, Switch13/2, Switch12/2, Switch11/2, Switch10/2
  Relational Operator3/1 -> Switch21/2, Switch19/2, Switch18/2, Switch17/2, Switch16/2, Switch15/2
  Relational Operator4/1 -> Switch28/2, Switch26/2, Switch25/2, Switch24/2, Switch23/2, Switch22/2
  Relational Operator5/1 -> Switch35/2, Switch33/2, Switch32/2, Switch31/2, Switch30/2, Switch29/2
  Relational Operator6/1 -> Switch42/2, Switch40/2, Switch39/2, Switch38/2, Switch37/2, Switch36/2
  Relational Operator7/1 -> Switch49/2, Switch47/2, Switch46/2, Switch45/2, Switch44/2, Switch43/2
  Relational Operator8/1 -> Switch56/2, Switch54/2, Switch53/2, Switch52/2, Switch51/2, Switch50/2
  Relational Operator9/1 -> Switch63/2, Switch61/2, Switch60/2, Switch59/2, Switch58/2, Switch57/2
  Switch/1 -> Relational Operator/2
  Switch1/1 -> Delay/1
  Switch10/1 -> Delay26/1, MATLAB Function/5(Index_2)
  Switch100/1 -> mux6/1, Delay337/1
  Switch101/1 -> mux6/2, Delay341/1
  Switch102/1 -> mux6/3, Delay342/1
  Switch103/1 -> mux6/4, Delay343/1
  Switch104/1 -> Relational Operator15/2
  Switch105/1 -> Delay325/1
  Switch106/1 -> Delay349/1, MATLAB Function/47(Index_16)
  Switch107/1 -> mux7/1, Delay360/1
  Switch108/1 -> mux7/2, Delay364/1
  Switch109/1 -> mux7/3, Delay365/1
  Switch11/1 -> mux1/1, Delay37/1
  Switch110/1 -> mux7/4, Delay366/1
  Switch111/1 -> Relational Operator16/2
  Switch112/1 -> Delay348/1
  Switch12/1 -> mux1/2, Delay41/1
  Switch13/1 -> mux1/3, Delay42/1
  Switch14/1 -> mux1/4, Delay43/1
  Switch15/1 -> Delay50/1, MATLAB Function/8(Index_3)
  Switch16/1 -> mux8/1, Delay61/1
  Switch17/1 -> mux8/2, Delay65/1
  Switch18/1 -> mux8/3, Delay66/1
  Switch19/1 -> mux8/4, Delay67/1
  Switch2/1 -> Delay1/1, MATLAB Function/2(Index_1)
  Switch20/1 -> Relational Operator3/2
  Switch21/1 -> Delay49/1
  Switch22/1 -> Delay73/1, MATLAB Function/11(Index_4)
  Switch23/1 -> mux9/1, Delay84/1
  Switch24/1 -> mux9/2, Delay88/1
  Switch25/1 -> mux9/3, Delay89/1
  Switch26/1 -> mux9/4, Delay90/1
  Switch27/1 -> Relational Operator4/2
  Switch28/1 -> Delay72/1
  Switch29/1 -> Delay96/1, MATLAB Function/14(Index_5)
  Switch3/1 -> mux/1, Delay2/1
  Switch30/1 -> mux10/1, Delay107/1
  Switch31/1 -> mux10/2, Delay111/1
  Switch32/1 -> mux10/3, Delay112/1
  Switch33/1 -> mux10/4, Delay113/1
  Switch34/1 -> Relational Operator5/2
  Switch35/1 -> Delay95/1
  Switch36/1 -> Delay119/1, MATLAB Function/17(Index_6)
  Switch37/1 -> mux11/1, Delay130/1
  Switch38/1 -> mux11/2, Delay134/1
  Switch39/1 -> mux11/3, Delay135/1
  Switch4/1 -> mux/2, Delay3/1
  Switch40/1 -> mux11/4, Delay136/1
  Switch41/1 -> Relational Operator6/2
  Switch42/1 -> Delay118/1
  Switch43/1 -> Delay142/1, MATLAB Function/20(Index_7)
  Switch44/1 -> mux12/1, Delay153/1
  Switch45/1 -> mux12/2, Delay157/1
  Switch46/1 -> mux12/3, Delay158/1
  Switch47/1 -> mux12/4, Delay159/1
  Switch48/1 -> Relational Operator7/2
  Switch49/1 -> Delay141/1
  Switch5/1 -> mux/3, Delay4/1
  Switch50/1 -> Delay165/1, MATLAB Function/23(Index_8)
  Switch51/1 -> mux13/1, Delay176/1
  Switch52/1 -> mux13/2, Delay180/1
  Switch53/1 -> mux13/3, Delay181/1
  Switch54/1 -> mux13/4, Delay182/1
  Switch55/1 -> Relational Operator8/2
  Switch56/1 -> Delay164/1
  Switch57/1 -> Delay275/1, MATLAB Function/26(Index_9)
  Switch58/1 -> mux14/1, Delay286/1
  Switch59/1 -> mux14/2, Delay290/1
  Switch6/1 -> mux/4, Delay5/1
  Switch60/1 -> mux14/3, Delay291/1
  Switch61/1 -> mux14/4, Delay292/1
  Switch62/1 -> Relational Operator9/2
  Switch63/1 -> Delay274/1
  Switch64/1 -> Delay298/1, MATLAB Function/29(Index_10)
  Switch65/1 -> mux15/1, Delay194/1
  Switch66/1 -> mux15/2, Delay198/1
  Switch67/1 -> mux15/3, Delay199/1
  Switch68/1 -> mux15/4, Delay200/1
  Switch69/1 -> Relational Operator10/2
  Switch7/1 -> done/1
  Switch70/1 -> Delay297/1
  Switch71/1 -> Delay206/1, MATLAB Function/32(Index_11)
  Switch72/1 -> mux2/1, Delay217/1
  Switch73/1 -> mux2/2, Delay221/1
  Switch74/1 -> mux2/3, Delay222/1
  Switch75/1 -> mux2/4, Delay223/1
  Switch76/1 -> Relational Operator11/2
  Switch77/1 -> Delay205/1
  Switch78/1 -> Delay229/1, MATLAB Function/35(Index_12)
  Switch79/1 -> mux3/1, Delay240/1
  Switch8/1 -> Relational Operator2/2
  Switch80/1 -> mux3/2, Delay244/1
  Switch81/1 -> mux3/3, Delay245/1
  Switch82/1 -> mux3/4, Delay246/1
  Switch83/1 -> Relational Operator12/2
  Switch84/1 -> Delay228/1
  Switch85/1 -> Delay252/1, MATLAB Function/38(Index_13)
  Switch86/1 -> mux4/1, Delay263/1
  Switch87/1 -> mux4/2, Delay267/1
  Switch88/1 -> mux4/3, Delay268/1
  Switch89/1 -> mux4/4, Delay269/1
  Switch9/1 -> Delay25/1
  Switch90/1 -> Relational Operator13/2
  Switch91/1 -> Delay251/1
  Switch92/1 -> Delay303/1, MATLAB Function/41(Index_14)
  Switch93/1 -> mux5/1, Delay314/1
  Switch94/1 -> mux5/2, Delay318/1
  Switch95/1 -> mux5/3, Delay319/1
  Switch96/1 -> mux5/4, Delay320/1
  Switch97/1 -> Relational Operator14/2
  Switch98/1 -> Delay302/1
  Switch99/1 -> Delay326/1, MATLAB Function/44(Index_15)
  Switch_on1/1 -> Switch2/1, Relational Operator1/2, Delay18/1, Compare To Constant/1(u)
  Switch_on10/1 -> Switch9/1, Relational Operator2/1, Delay34/1
  Switch_on100/1 -> Delay373/1, MinMax/3
  Switch_on101/1 -> Delay374/1, MinMax/4
  Switch_on102/1 -> Delay377/1, MinMax/7
  Switch_on103/1 -> Delay378/1, MinMax/8
  Switch_on104/1 -> Delay375/1, MinMax/5
  Switch_on105/1 -> Delay376/1, MinMax/6
  Switch_on106/1 -> Delay381/1, MinMax/11
  Switch_on107/1 -> Delay382/1, MinMax/12
  Switch_on108/1 -> Delay379/1, MinMax/9
  Switch_on109/1 -> Delay380/1, MinMax/10
  Switch_on11/1 -> Switch13/1, Delay39/1
  Switch_on110/1 -> Delay385/1, MinMax/15
  Switch_on111/1 -> Delay386/1, MinMax/16
  Switch_on112/1 -> Delay383/1, MinMax/13
  Switch_on113/1 -> Delay384/1, MinMax/14
  Switch_on12/1 -> Switch14/1, Delay40/1
  Switch_on14/1 -> Switch21/1, Relational Operator3/1, Delay58/1
  Switch_on15/1 -> Switch18/1, Delay63/1
  Switch_on16/1 -> Switch19/1, Delay64/1
  Switch_on17/1 -> Switch15/1, Delay59/1, Compare To Constant2/1(u)
  Switch_on18/1 -> Switch16/1, Delay60/1
  Switch_on19/1 -> Switch17/1, Delay62/1
  Switch_on2/1 -> Switch3/1, Delay19/1
  Switch_on20/1 -> Switch28/1, Relational Operator4/1, Delay81/1
  Switch_on21/1 -> Switch25/1, Delay86/1
  Switch_on22/1 -> Switch26/1, Delay87/1
  Switch_on23/1 -> Switch22/1, Delay82/1, Compare To Constant3/1(u)
  Switch_on24/1 -> Switch23/1, Delay83/1
  Switch_on25/1 -> Switch24/1, Delay85/1
  Switch_on26/1 -> Switch35/1, Relational Operator5/1, Delay104/1
  Switch_on27/1 -> Switch32/1, Delay109/1
  Switch_on28/1 -> Switch33/1, Delay110/1
  Switch_on29/1 -> Switch29/1, Delay105/1, Compare To Constant4/1(u)
  Switch_on3/1 -> Switch4/1, Delay20/1
  Switch_on30/1 -> Switch30/1, Delay106/1
  Switch_on31/1 -> Switch31/1, Delay108/1
  Switch_on32/1 -> Switch42/1, Relational Operator6/1, Delay127/1
  Switch_on33/1 -> Switch39/1, Delay132/1
  Switch_on34/1 -> Switch40/1, Delay133/1
  Switch_on35/1 -> Switch36/1, Delay128/1, Compare To Constant5/1(u)
  Switch_on36/1 -> Switch37/1, Delay129/1
  Switch_on37/1 -> Switch38/1, Delay131/1
  Switch_on38/1 -> Switch49/1, Relational Operator7/1, Delay150/1
  Switch_on39/1 -> Switch46/1, Delay155/1
  Switch_on4/1 -> Switch1/1, Relational Operator/1, Delay17/1
  Switch_on40/1 -> Switch47/1, Delay156/1
  Switch_on41/1 -> Switch43/1, Delay151/1, Compare To Constant6/1(u)
  Switch_on42/1 -> Switch44/1, Delay152/1
  Switch_on43/1 -> Switch45/1, Delay154/1
  Switch_on44/1 -> Switch56/1, Relational Operator8/1, Delay173/1
  Switch_on45/1 -> Switch53/1, Delay178/1
  Switch_on46/1 -> Switch54/1, Delay179/1
  Switch_on47/1 -> Switch50/1, Delay174/1, Compare To Constant7/1(u)
  Switch_on48/1 -> Switch51/1, Delay175/1
  Switch_on49/1 -> Switch52/1, Delay177/1
  Switch_on5/1 -> Switch5/1, Delay21/1
  Switch_on50/1 -> Switch63/1, Relational Operator9/1, Delay283/1
  Switch_on51/1 -> Switch60/1, Delay288/1
  Switch_on52/1 -> Switch61/1, Delay289/1
  Switch_on53/1 -> Switch57/1, Delay284/1, Compare To Constant8/1(u)
  Switch_on54/1 -> Switch58/1, Delay285/1
  Switch_on55/1 -> Switch59/1, Delay287/1
  Switch_on56/1 -> Switch70/1, Relational Operator10/1, Delay191/1
  Switch_on57/1 -> Switch67/1, Delay196/1
  Switch_on58/1 -> Switch68/1, Delay197/1
  Switch_on59/1 -> Switch64/1, Delay192/1, Compare To Constant9/1(u)
  Switch_on6/1 -> Switch6/1, Delay22/1
  Switch_on60/1 -> Switch65/1, Delay193/1
  Switch_on61/1 -> Switch66/1, Delay195/1
  Switch_on62/1 -> Switch77/1, Relational Operator11/1, Delay214/1
  Switch_on63/1 -> Switch74/1, Delay219/1
  Switch_on64/1 -> Switch75/1, Delay220/1
  Switch_on65/1 -> Switch71/1, Delay215/1, Compare To Constant10/1(u)
  Switch_on66/1 -> Switch72/1, Delay216/1
  Switch_on67/1 -> Switch73/1, Delay218/1
  Switch_on68/1 -> Switch84/1, Relational Operator12/1, Delay237/1
  Switch_on69/1 -> Switch81/1, Delay242/1
  Switch_on7/1 -> Switch10/1, Delay35/1, Compare To Constant1/1(u)
  Switch_on70/1 -> Switch82/1, Delay243/1
  Switch_on71/1 -> Switch78/1, Delay238/1, Compare To Constant11/1(u)
  Switch_on72/1 -> Switch79/1, Delay239/1
  Switch_on73/1 -> Switch80/1, Delay241/1
  Switch_on74/1 -> Switch91/1, Relational Operator13/1, Delay260/1
  Switch_on75/1 -> Switch88/1, Delay265/1
  Switch_on76/1 -> Switch89/1, Delay266/1
  Switch_on77/1 -> Switch85/1, Delay261/1, Compare To Constant12/1(u)
  Switch_on78/1 -> Switch86/1, Delay262/1
  Switch_on79/1 -> Switch87/1, Delay264/1
  Switch_on8/1 -> Switch11/1, Delay36/1
  Switch_on80/1 -> Switch98/1, Relational Operator14/1, Delay311/1
  Switch_on81/1 -> Switch95/1, Delay316/1
  Switch_on82/1 -> Switch96/1, Delay317/1
  Switch_on83/1 -> Switch92/1, Delay312/1, Compare To Constant13/1(u)
  Switch_on84/1 -> Switch93/1, Delay313/1
  Switch_on85/1 -> Switch94/1, Delay315/1
  Switch_on86/1 -> Switch105/1, Relational Operator15/1, Delay334/1
  Switch_on87/1 -> Switch102/1, Delay339/1
  Switch_on88/1 -> Switch103/1, Delay340/1
  Switch_on89/1 -> Switch99/1, Delay335/1, Compare To Constant14/1(u)
  Switch_on9/1 -> Switch12/1, Delay38/1
  Switch_on90/1 -> Switch100/1, Delay336/1
  Switch_on91/1 -> Switch101/1, Delay338/1
  Switch_on92/1 -> Switch112/1, Relational Operator16/1, Delay357/1
  Switch_on93/1 -> Switch109/1, Delay362/1
  Switch_on94/1 -> Switch110/1, Delay363/1
  Switch_on95/1 -> Switch106/1, Delay358/1, Compare To Constant15/1(u)
  Switch_on96/1 -> Switch107/1, Delay359/1
  Switch_on97/1 -> Switch108/1, Delay361/1
  Switch_on98/1 -> Delay371/1, MinMax/1
  Switch_on99/1 -> Delay372/1, MinMax/2
  t/1 -> Delay7_out1_0_wire/1
  t/2 -> Delay7_out1_1_wire/1
  t/3 -> Delay7_out1_2_wire/1
  t/4 -> Delay7_out1_3_wire/1
  t/5 -> Delay7_out1_4_wire/1
  t/6 -> Delay7_out1_5_wire/1
  t/7 -> Delay7_out1_6_wire/1
  t/8 -> Delay7_out1_7_wire/1
  t/9 -> Delay7_out1_8_wire/1
  t/10 -> Delay7_out1_9_wire/1
  t/11 -> Delay7_out1_10_wire/1
  t/12 -> Delay7_out1_11_wire/1
  t/13 -> Delay7_out1_12_wire/1
  t/14 -> Delay7_out1_13_wire/1
  t/15 -> Delay7_out1_14_wire/1
  t/16 -> Delay7_out1_15_wire/1
  t1/1 -> Delay16_out1_0_wire/1
  t1/2 -> Delay16_out1_1_wire/1
  t1/3 -> Delay16_out1_2_wire/1
  t1/4 -> Delay16_out1_3_wire/1
  t1/5 -> Delay16_out1_4_wire/1
  t1/6 -> Delay16_out1_5_wire/1
  t1/7 -> Delay16_out1_6_wire/1
  t1/8 -> Delay16_out1_7_wire/1
  t1/9 -> Delay16_out1_8_wire/1
  t1/10 -> Delay16_out1_9_wire/1
  t1/11 -> Delay16_out1_10_wire/1
  t1/12 -> Delay16_out1_11_wire/1
  t1/13 -> Delay16_out1_12_wire/1
  t1/14 -> Delay16_out1_13_wire/1
  t1/15 -> Delay16_out1_14_wire/1
  t1/16 -> Delay16_out1_15_wire/1
  t1/17 -> Delay16_out1_16_wire/1
  t1/18 -> Delay16_out1_17_wire/1
  t1/19 -> Delay16_out1_18_wire/1
  t1/20 -> Delay16_out1_19_wire/1
  t1/21 -> Delay16_out1_20_wire/1
  t1/22 -> Delay16_out1_21_wire/1
  t1/23 -> Delay16_out1_22_wire/1
  t1/24 -> Delay16_out1_23_wire/1
  t1/25 -> Delay16_out1_24_wire/1
  t1/26 -> Delay16_out1_25_wire/1
  t1/27 -> Delay16_out1_26_wire/1
  t1/28 -> Delay16_out1_27_wire/1
  t1/29 -> Delay16_out1_28_wire/1
  t1/30 -> Delay16_out1_29_wire/1
  t1/31 -> Delay16_out1_30_wire/1
  t1/32 -> Delay16_out1_31_wire/1
  t1/33 -> Delay16_out1_32_wire/1
  t1/34 -> Delay16_out1_33_wire/1
  t1/35 -> Delay16_out1_34_wire/1
  t1/36 -> Delay16_out1_35_wire/1
  t1/37 -> Delay16_out1_36_wire/1
  t1/38 -> Delay16_out1_37_wire/1
  t1/39 -> Delay16_out1_38_wire/1
  t1/40 -> Delay16_out1_39_wire/1
  t1/41 -> Delay16_out1_40_wire/1
  t1/42 -> Delay16_out1_41_wire/1
  t1/43 -> Delay16_out1_42_wire/1
  t1/44 -> Delay16_out1_43_wire/1
  t1/45 -> Delay16_out1_44_wire/1
  t1/46 -> Delay16_out1_45_wire/1
  t1/47 -> Delay16_out1_46_wire/1
  t1/48 -> Delay16_out1_47_wire/1
  t1/49 -> Delay16_out1_48_wire/1
  t1/50 -> Delay16_out1_49_wire/1
  t1/51 -> Delay16_out1_50_wire/1
  t1/52 -> Delay16_out1_51_wire/1
  t1/53 -> Delay16_out1_52_wire/1
  t1/54 -> Delay16_out1_53_wire/1
  t1/55 -> Delay16_out1_54_wire/1
  t1/56 -> Delay16_out1_55_wire/1
  t1/57 -> Delay16_out1_56_wire/1
  t1/58 -> Delay16_out1_57_wire/1
  t1/59 -> Delay16_out1_58_wire/1
  t1/60 -> Delay16_out1_59_wire/1
  t1/61 -> Delay16_out1_60_wire/1
  t1/62 -> Delay16_out1_61_wire/1
  t1/63 -> Delay16_out1_62_wire/1
  t1/64 -> Delay16_out1_63_wire/1
